simulink model "SeparatelyexcitedDCmotorFANS"  (R2021a)
settings: Solver=VariableStepAuto  StartTime=0.0  StopTime=10.0  RelTol=1e-3
settings Model: Creator=ygxdy  LastModifiedBy=ygxdy

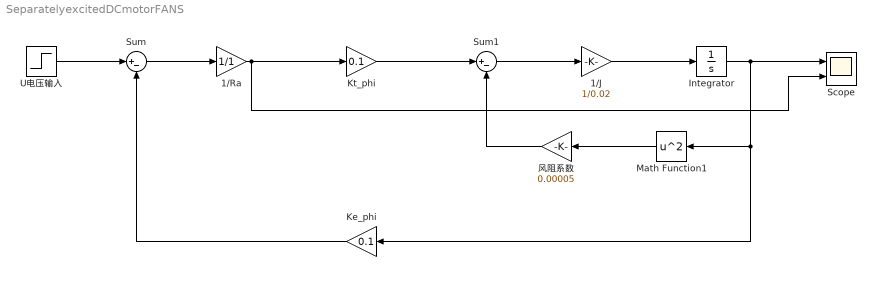
== system SeparatelyexcitedDCmotorFANS ==
  1/J : Gain  Gain=1/0.02
  1/Ra : Gain  Gain=1/1
  Integrator : Integrator
  Ke_phi : Gain  Gain=0.1
  Kt_phi : Gain  Gain=0.1
  Math Function1 : Math  Operator=square  SaturateOnIntegerOverflow=on
  Scope : Scope  NumInputPorts=2
  Sum : Sum  Inputs=|+-
  Sum1 : Sum  Inputs=|+-
  U电压输入 : Step  Time=0  After=24  SampleTime=0
  风阻系数 : Gain  Gain=0.00005
  wires:
  U电压输入/1 -> Sum/1
  Sum/1 -> 1/Ra/1
  1/Ra/1 -> Scope/2, Kt_phi/1
  Kt_phi/1 -> Sum1/1
  Sum1/1 -> 1/J/1
  1/J/1 -> Integrator/1
  Integrator/1 -> Scope/1, Math Function1/1, Ke_phi/1
  Ke_phi/1 -> Sum/2
  风阻系数/1 -> Sum1/2
  Math Function1/1 -> 风阻系数/1
